simulink model "CompleteModelSimulink"  (R2024a)
settings: Solver=ode45  StartTime=0.0  StopTime=endtime  RelTol=1e-3
values from neighbouring files (symbols this model uses):
  D = 0.069    [CompleteModel.m]
  D_H = 2    [PID_Current.m]    (also in PID_NoCurrent.m = 1)
  D_X = 2    [PID_Current.m]    (also in PID_NoCurrent.m = 1.05)
  D_Y = 2    [PID_Current.m]    (also in PID_NoCurrent.m = 0.8)
  DC =     [DC.mat]
  I_H = 0.1    [PID_Current.m]    (also in PID_NoCurrent.m = 0.01)
  I_X = 0.1    [PID_Current.m]    (also in PID_NoCurrent.m = 0.001)
  I_Y = 0.2    [PID_Current.m]    (also in PID_NoCurrent.m = 0.01)
  InitialPos = [0;0;0]    [CompleteModel.m]
  M_matrix = [2.5 0 0; 0 2.50 0; 0 0 1]    [CompleteModel.m]
  P_H = 2    [PID_Current.m]    (also in PID_NoCurrent.m = 1)
  P_X = 2    [PID_Current.m]    (also in PID_NoCurrent.m = 0.75)
  P_Y = 2    [PID_Current.m]    (also in PID_NoCurrent.m = 1.3)
  Ref = [1;0;0]    [CompleteModel.m]
  SpeedFactor = 0.07    [CompleteModel.m]
  SR =     [SR.mat]
  T_matrix = [0 1 0; 1 0 1; 0.35 -0.065 -0.35]    [CompleteModel.m]
  TauE = [-0.15;0;0]    [CompleteModel.m]
libraries: slpidlib x8
(part 2 of 2)

== system CompleteModelSimulink/Starboard Azimith Thrust generation/Motor+Control SB/Current Controller ==
  Ia : Inport
  Ia ref* : Inport  Port=2
  Constant : Constant  Value=DC.Irated
  Divide : Product  Inputs=*/
  Error : Sum  Inputs=|+-
  PID Controller : slpidlib/PID Controller  Controller=PID  Form=Ideal  TimeDomain=Continuous-time  UseExternalTs=off  SampleTime=-1  IntegratorMethod=Forward Euler  FilterMethod=Forward Euler  ControllerParametersSource=internal  P=7.2353580328522  I=2.78600690342995  UseKiTs=off  D=0.0824758010540437  UseExternalDerivativeSource=off  N=135.726193036092  UseFilter=on  TunerSelectOption=Transfer Function Based (PID Tuner App)  InitialConditionSource=internal  InitialConditionForIntegrator=0  InitialConditionForFilter=0  DifferentiatorICPrevScaledInput=0  ExternalReset=none  TrackingMode=off  Kt=1  LimitOutput=off  SatLimitsSource=internal  UpperSaturationLimit=inf  LowerSaturationLimit=-inf  LinearizeAsGain=on  AntiWindupMode=none  Kb=1  LimitIntegrator=off  UpperIntegratorSaturationLimit=inf  LowerIntegratorSaturationLimit=-inf  POutMin=[]  POutMax=[]  IOutMin=[]  IOutMax=[]  DOutMin=[]  DOutMax=[]  NOutMin=[]  NOutMax=[]  SumOutMin=[]  SumOutMax=[]  SaturationOutMin=[]  SaturationOutMax=[]  PParamMin=[]  PParamMax=[]  IParamMin=[]  IParamMax=[]  DParamMin=[]  DParamMax=[]  NParamMin=[]  NParamMax=[]  KbParamMin=[]  KbParamMax=[]  KtParamMin=[]  KtParamMax=[]  KbOutMin=[]  KbOutMax=[]  KtOutMin=[]  KtOutMax=[]  IntegratorOutMin=[]  IntegratorOutMax=[]  FilterOutMin=[]  FilterOutMax=[]  SumI1OutMin=[]  SumI1OutMax=[]  SumI2OutMin=[]  SumI2OutMax=[]  SumI3OutMin=[]  SumI3OutMax=[]  SumI4OutMin=[]  SumI4OutMax=[]  SumDOutMin=[]  SumDOutMax=[]  DifferentiatorOutMin=[]  DifferentiatorOutMax=[]  FilterDiffOutCoefMin=[]  FilterDiffOutCoefMax=[]  ReciprocalOutMin=[]  ReciprocalOutMax=[]  SumDenOutMin=[]  SumDenOutMax=[]  SumNumOutMin=[]  SumNumOutMax=[]  DivideOutMin=[]  DivideOutMax=[]  UdiffTsProdOutMin=[]  UdiffTsProdOutMax=[]  NTsProdOutMin=[]  NTsProdOutMax=[]  UintegralTsProdOutMin=[]  UintegralTsProdOutMax=[]  UngainTsProdOutMin=[]  UngainTsProdOutMax=[]  ClampingZeroOutDataTypeStr=Inherit: Inherit via back propagation  ClampingZeroOutMin=[]  ClampingZeroOutMax=[]  FilterDenConstantOutDataTypeStr=Inherit: Inherit via back propagation  FilterDenConstantOutMin=[]  FilterDenConstantOutMax=[]  PCopyOutDataTypeStr=Inherit: Inherit via back propagation  PCopyOutMin=[]  PCopyOutMax=[]  NCopyOutDataTypeStr=Inherit: Inherit via back propagation  NCopyOutMin=[]  NCopyOutMax=[]  IntegratorContinuousStateAttributes=''  IntegratorStateMustResolveToSignalObject=off  IntegratorRTWStateStorageClass=Auto  FilterContinuousStateAttributes=''  FilterStateMustResolveToSignalObject=off  FilterRTWStateStorageClass=Auto  ParallelPVariant=Passthrough  IdealPVariant=InternalParameters  IVariant=InternalParameters  DVariant=InternalParameters  IntegratorVariant=Continuous  SatVariant=Disabled  AWVariant=Passthrough  PCopyVariant=Disabled  TRVariant=Disabled  FdbkBlocksVariant=Forward  IdealPFdbkVariant=Disabled  SatFdbkVariant=Disabled  DerivativeFilterVariant=ContFilter  NVariant=InternalParameters  NCopyVariant=Disabled  FilterICVariant=InternalICsFilter  IntegratorICVariant=InternalICs  ExternalResetVariant=Disabled  TRSumVariant=Passthrough  SumFdbkVariant=Disabled  SumVariant=Sum_PID  TsampFilterVariant=InternalTs  TsampNgainVariant=Passthrough  TsampIntegralVariant=Disabled_SignalSpec  ExternalSaturationOutDataTypeStr=Inherit: Same as second input  DerivativeSourceVariant=ErrorSignal
  PID Controller1 : slpidlib/PID Controller  Commented=on  Controller=PID  Form=Ideal  TimeDomain=Continuous-time  UseExternalTs=off  SampleTime=-1  IntegratorMethod=Forward Euler  FilterMethod=Forward Euler  ControllerParametersSource=internal  P=7.2353580328522  I=2.78600690342995  UseKiTs=off  D=0.0824758010540437  UseExternalDerivativeSource=off  N=135.726193036092  UseFilter=on  TunerSelectOption=Transfer Function Based (PID Tuner App)  InitialConditionSource=internal  InitialConditionForIntegrator=0  InitialConditionForFilter=0  DifferentiatorICPrevScaledInput=0  ExternalReset=none  TrackingMode=off  Kt=1  LimitOutput=off  SatLimitsSource=internal  UpperSaturationLimit=inf  LowerSaturationLimit=-inf  LinearizeAsGain=on  AntiWindupMode=none  Kb=1  LimitIntegrator=off  UpperIntegratorSaturationLimit=inf  LowerIntegratorSaturationLimit=-inf  POutMin=[]  POutMax=[]  IOutMin=[]  IOutMax=[]  DOutMin=[]  DOutMax=[]  NOutMin=[]  NOutMax=[]  SumOutMin=[]  SumOutMax=[]  SaturationOutMin=[]  SaturationOutMax=[]  PParamMin=[]  PParamMax=[]  IParamMin=[]  IParamMax=[]  DParamMin=[]  DParamMax=[]  NParamMin=[]  NParamMax=[]  KbParamMin=[]  KbParamMax=[]  KtParamMin=[]  KtParamMax=[]  KbOutMin=[]  KbOutMax=[]  KtOutMin=[]  KtOutMax=[]  IntegratorOutMin=[]  IntegratorOutMax=[]  FilterOutMin=[]  FilterOutMax=[]  SumI1OutMin=[]  SumI1OutMax=[]  SumI2OutMin=[]  SumI2OutMax=[]  SumI3OutMin=[]  SumI3OutMax=[]  SumI4OutMin=[]  SumI4OutMax=[]  SumDOutMin=[]  SumDOutMax=[]  DifferentiatorOutMin=[]  DifferentiatorOutMax=[]  FilterDiffOutCoefMin=[]  FilterDiffOutCoefMax=[]  ReciprocalOutMin=[]  ReciprocalOutMax=[]  SumDenOutMin=[]  SumDenOutMax=[]  SumNumOutMin=[]  SumNumOutMax=[]  DivideOutMin=[]  DivideOutMax=[]  UdiffTsProdOutMin=[]  UdiffTsProdOutMax=[]  NTsProdOutMin=[]  NTsProdOutMax=[]  UintegralTsProdOutMin=[]  UintegralTsProdOutMax=[]  UngainTsProdOutMin=[]  UngainTsProdOutMax=[]  ClampingZeroOutDataTypeStr=Inherit: Inherit via back propagation  ClampingZeroOutMin=[]  ClampingZeroOutMax=[]  FilterDenConstantOutDataTypeStr=Inherit: Inherit via back propagation  FilterDenConstantOutMin=[]  FilterDenConstantOutMax=[]  PCopyOutDataTypeStr=Inherit: Inherit via back propagation  PCopyOutMin=[]  PCopyOutMax=[]  NCopyOutDataTypeStr=Inherit: Inherit via back propagation  NCopyOutMin=[]  NCopyOutMax=[]  IntegratorContinuousStateAttributes=''  IntegratorStateMustResolveToSignalObject=off  IntegratorRTWStateStorageClass=Auto  FilterContinuousStateAttributes=''  FilterStateMustResolveToSignalObject=off  FilterRTWStateStorageClass=Auto  ParallelPVariant=Passthrough  IdealPVariant=InternalParameters  IVariant=InternalParameters  DVariant=InternalParameters  IntegratorVariant=Continuous  SatVariant=Disabled  AWVariant=Passthrough  PCopyVariant=Disabled  TRVariant=Disabled  FdbkBlocksVariant=Forward  IdealPFdbkVariant=Disabled  SatFdbkVariant=Disabled  DerivativeFilterVariant=ContFilter  NVariant=InternalParameters  NCopyVariant=Disabled  FilterICVariant=InternalICsFilter  IntegratorICVariant=InternalICs  ExternalResetVariant=Disabled  TRSumVariant=Passthrough  SumFdbkVariant=Disabled  SumVariant=Sum_PID  TsampFilterVariant=InternalTs  TsampNgainVariant=Passthrough  TsampIntegralVariant=Disabled_SignalSpec  ExternalSaturationOutDataTypeStr=Inherit: Same as second input  DerivativeSourceVariant=ErrorSignal
  Saturation : Saturate  UpperLimit=1.2*DC.Irated  LowerLimit=-0.5*DC.Irated
  Ia ref : Outport
  wires:
  Error/1 -> Divide/1
  Divide/1 -> PID Controller/1
  PID Controller/1 -> Saturation/1
  Ia/1 -> Error/2
  Saturation/1 -> Ia ref/1
  Ia ref*/1 -> Error/1
  Constant/1 -> Divide/2

== system CompleteModelSimulink/Starboard Azimith Thrust generation/Motor+Control SB/Motor system ==
  Terminal Voltage : Inport
  Mechnical Torque : Inport  Port=2
  Electrical Equation : Subsystem
  Mechnical Equation : Subsystem
  Ia : Outport
  Wm1 : Outport  Port=2
  wires:
  Electrical Equation/1(Ia) -> Ia/1, Mechnical Equation/1(Ia)
  Mechnical Torque/1 -> Mechnical Equation/2(Mechnical Torque)
  Terminal Voltage/1 -> Electrical Equation/1(Terminal Voltage)
  Mechnical Equation/1(Wm) -> Wm1/1, Electrical Equation/2(Wm)

== system CompleteModelSimulink/Starboard Azimith Thrust generation/Motor+Control SB/Speed control ==
  Ref speed : Inport
  Act speed : Inport  Port=2
  Constant : Constant  Value=DC.Omegarated
  Divide : Product  Inputs=/*
  PID Controller2 : slpidlib/PID Controller  Controller=PID  Form=Ideal  TimeDomain=Continuous-time  UseExternalTs=off  SampleTime=-1  IntegratorMethod=Forward Euler  FilterMethod=Forward Euler  ControllerParametersSource=internal  P=301.958567368747  I=2.49617195964231  UseKiTs=off  D=0.0354093832005891  UseExternalDerivativeSource=off  N=1725.20945072566  UseFilter=on  TunerSelectOption=Transfer Function Based (PID Tuner App)  InitialConditionSource=internal  InitialConditionForIntegrator=0  InitialConditionForFilter=0  DifferentiatorICPrevScaledInput=0  ExternalReset=none  TrackingMode=off  Kt=1  LimitOutput=off  SatLimitsSource=internal  UpperSaturationLimit=inf  LowerSaturationLimit=-inf  LinearizeAsGain=on  AntiWindupMode=none  Kb=1  LimitIntegrator=off  UpperIntegratorSaturationLimit=inf  LowerIntegratorSaturationLimit=-inf  POutMin=[]  POutMax=[]  IOutMin=[]  IOutMax=[]  DOutMin=[]  DOutMax=[]  NOutMin=[]  NOutMax=[]  SumOutMin=[]  SumOutMax=[]  SaturationOutMin=[]  SaturationOutMax=[]  PParamMin=[]  PParamMax=[]  IParamMin=[]  IParamMax=[]  DParamMin=[]  DParamMax=[]  NParamMin=[]  NParamMax=[]  KbParamMin=[]  KbParamMax=[]  KtParamMin=[]  KtParamMax=[]  KbOutMin=[]  KbOutMax=[]  KtOutMin=[]  KtOutMax=[]  IntegratorOutMin=[]  IntegratorOutMax=[]  FilterOutMin=[]  FilterOutMax=[]  SumI1OutMin=[]  SumI1OutMax=[]  SumI2OutMin=[]  SumI2OutMax=[]  SumI3OutMin=[]  SumI3OutMax=[]  SumI4OutMin=[]  SumI4OutMax=[]  SumDOutMin=[]  SumDOutMax=[]  DifferentiatorOutMin=[]  DifferentiatorOutMax=[]  FilterDiffOutCoefMin=[]  FilterDiffOutCoefMax=[]  ReciprocalOutMin=[]  ReciprocalOutMax=[]  SumDenOutMin=[]  SumDenOutMax=[]  SumNumOutMin=[]  SumNumOutMax=[]  DivideOutMin=[]  DivideOutMax=[]  UdiffTsProdOutMin=[]  UdiffTsProdOutMax=[]  NTsProdOutMin=[]  NTsProdOutMax=[]  UintegralTsProdOutMin=[]  UintegralTsProdOutMax=[]  UngainTsProdOutMin=[]  UngainTsProdOutMax=[]  ClampingZeroOutDataTypeStr=Inherit: Inherit via back propagation  ClampingZeroOutMin=[]  ClampingZeroOutMax=[]  FilterDenConstantOutDataTypeStr=Inherit: Inherit via back propagation  FilterDenConstantOutMin=[]  FilterDenConstantOutMax=[]  PCopyOutDataTypeStr=Inherit: Inherit via back propagation  PCopyOutMin=[]  PCopyOutMax=[]  NCopyOutDataTypeStr=Inherit: Inherit via back propagation  NCopyOutMin=[]  NCopyOutMax=[]  IntegratorContinuousStateAttributes=''  IntegratorStateMustResolveToSignalObject=off  IntegratorRTWStateStorageClass=Auto  FilterContinuousStateAttributes=''  FilterStateMustResolveToSignalObject=off  FilterRTWStateStorageClass=Auto  ParallelPVariant=Passthrough  IdealPVariant=InternalParameters  IVariant=InternalParameters  DVariant=InternalParameters  IntegratorVariant=Continuous  SatVariant=Disabled  AWVariant=Passthrough  PCopyVariant=Disabled  TRVariant=Disabled  FdbkBlocksVariant=Forward  IdealPFdbkVariant=Disabled  SatFdbkVariant=Disabled  DerivativeFilterVariant=ContFilter  NVariant=InternalParameters  NCopyVariant=Disabled  FilterICVariant=InternalICsFilter  IntegratorICVariant=InternalICs  ExternalResetVariant=Disabled  TRSumVariant=Passthrough  SumFdbkVariant=Disabled  SumVariant=Sum_PID  TsampFilterVariant=InternalTs  TsampNgainVariant=Passthrough  TsampIntegralVariant=Disabled_SignalSpec  ExternalSaturationOutDataTypeStr=Inherit: Same as second input  DerivativeSourceVariant=ErrorSignal
  Saturation : Saturate  UpperLimit=1.2*DC.Irated  LowerLimit=-0.5*DC.Irated
  Sum : Sum  Inputs=|+-
  Ia ref* : Outport
  wires:
  Saturation/1 -> Ia ref*/1
  PID Controller2/1 -> Saturation/1
  Divide/1 -> PID Controller2/1
  Ref speed/1 -> Sum/1
  Act speed/1 -> Sum/2
  Sum/1 -> Divide/2  "Error"
  Constant/1 -> Divide/1

== system CompleteModelSimulink/Vessel reaction to forces/Rotate local to global /Local to global x  ==
  X : Inport
  Y : Inport  Port=2
  theta : Inport  Port=3
  Add : Sum
  Product : Product
  Product1 : Product
  Trigonometric Function : Trigonometry  Operator=cos
  Trigonometric Function1 : Trigonometry
  x : Outport  VectorParamsAs1DForOutWhenUnconnected=off
  wires:
  Add/1 -> x/1
  Product1/1 -> Add/2
  Product/1 -> Add/1
  Y/1 -> Product1/1
  X/1 -> Product/1
  theta/1 -> Trigonometric Function1/1, Trigonometric Function/1
  Trigonometric Function1/1 -> Product1/2
  Trigonometric Function/1 -> Product/2

== system CompleteModelSimulink/Vessel reaction to forces/Rotate local to global /Local to global y ==
  X : Inport
  Y : Inport  Port=2
  theta : Inport  Port=3
  Product : Product
  Product1 : Product
  Sum : Sum  Inputs=-+
  Trigonometric Function : Trigonometry
  Trigonometric Function1 : Trigonometry  Operator=cos
  y : Outport  VectorParamsAs1DForOutWhenUnconnected=off
  wires:
  Sum/1 -> y/1
  Product1/1 -> Sum/2
  Y/1 -> Product1/1
  X/1 -> Product/1
  theta/1 -> Trigonometric Function1/1, Trigonometric Function/1
  Trigonometric Function1/1 -> Product1/2
  Trigonometric Function/1 -> Product/2
  Product/1 -> Sum/1

== system CompleteModelSimulink/Portside Azimuth Thrust generation/Motor+Control PS/Motor system/Electrical Equation ==
  Terminal Voltage : Inport
  Wm : Inport  Port=2
  I : Integrator
  Kt*wm : Gain  Gain=DC.Kb
  La*didt : Sum  Inputs=+--
  Ra*Ia : Gain  Gain=DC.Ra
  didt : Gain  Gain=1/DC.La
  Ia : Outport
  wires:
  Wm/1 -> Kt*wm/1
  Kt*wm/1 -> La*didt/2
  didt/1 -> I/1
  Terminal Voltage/1 -> La*didt/1
  La*didt/1 -> didt/1
  Ra*Ia/1 -> La*didt/3
  I/1 -> Ra*Ia/1, Ia/1

== system CompleteModelSimulink/Portside Azimuth Thrust generation/Motor+Control PS/Motor system/Mechnical Equation ==
  Ia : Inport
  Mechnical Torque : Inport  Port=2
  Cm*wm : Gain  Gain=DC.Cm
  Jm* dwdt : Sum  Inputs=-+-
  Kt*Ia : Gain  Gain=DC.Kt
  dwdt : Gain  Gain=1/DC.Jm
  wm : Integrator
  Wm : Outport
  wires:
  wm/1 -> Cm*wm/1, Wm/1
  dwdt/1 -> wm/1
  Mechnical Torque/1 -> Jm* dwdt/3
  Cm*wm/1 -> Jm* dwdt/1
  Jm* dwdt/1 -> dwdt/1
  Ia/1 -> Kt*Ia/1
  Kt*Ia/1 -> Jm* dwdt/2

== system CompleteModelSimulink/Starboard Azimith Thrust generation/Motor+Control SB/Motor system/Electrical Equation ==
  Terminal Voltage : Inport
  Wm : Inport  Port=2
  I : Integrator
  Kt*wm : Gain  Gain=DC.Kb
  La*didt : Sum  Inputs=+--
  Ra*Ia : Gain  Gain=DC.Ra
  didt : Gain  Gain=1/DC.La
  Ia : Outport
  wires:
  Wm/1 -> Kt*wm/1
  Kt*wm/1 -> La*didt/2
  didt/1 -> I/1
  Terminal Voltage/1 -> La*didt/1
  La*didt/1 -> didt/1
  Ra*Ia/1 -> La*didt/3
  I/1 -> Ra*Ia/1, Ia/1

== system CompleteModelSimulink/Starboard Azimith Thrust generation/Motor+Control SB/Motor system/Mechnical Equation ==
  Ia : Inport
  Mechnical Torque : Inport  Port=2
  Cm*wm : Gain  Gain=DC.Cm
  Jm* dwdt : Sum  Inputs=-+-
  Kt*Ia : Gain  Gain=DC.Kt
  dwdt : Gain  Gain=1/DC.Jm
  wm : Integrator
  Wm : Outport
  wires:
  wm/1 -> Cm*wm/1, Wm/1
  dwdt/1 -> wm/1
  Mechnical Torque/1 -> Jm* dwdt/3
  Cm*wm/1 -> Jm* dwdt/1
  Jm* dwdt/1 -> dwdt/1
  Ia/1 -> Kt*Ia/1
  Kt*Ia/1 -> Jm* dwdt/2

== matlab function CompleteModelSimulink/Vessel reaction to forces/Corriolis Matrix/MATLAB Function1 ==
  data: uv input; C output; Xudot input; Yvdot input; m input
function C = fcn(uv, Xudot, Yvdot, m)
a1 = Xudot*uv(1);
a2 = Yvdot*uv(2);

Ca = [0 0 a2; 0 0 -a1; -a2 a1 0];

Crb = [0 0 -m*uv(2); 0 0 m*uv(1); m*uv(2) -m*uv(1) 0];

C = Ca+Crb;

== matlab function CompleteModelSimulink/Vessel reaction to forces/Damping Vector/Damping ==
  data: uvr input; D output; X input; Y input; Yaw input; L input
function D = fcn(uvr, X, Y, Yaw, L)
    D11 = X(1)*uvr(1)^3+X(2)*uvr(1)^2+X(3)*uvr(1)+X(4);
    D22 = Y(1)*uvr(2)^3+Y(2)*uvr(2)^2+Y(3)*uvr(2)+Y(4);
    D33 = 1/80*Yaw(1)*uvr(3)^3*L^4+1/12*Yaw(2)*L^2*uvr(3);
D = [D11;D22;D33];

== matlab function CompleteModelSimulink/Portside Azimuth Thrust generation/Thrust to Torque/Matching PS ==
  data: Kt input; Kq output
function Kq = fcn(Kt)
coef = [-14.707 5.8681 -4.0985 1.5002];
J = coef(1)*Kt^3+coef(2)*Kt^2+coef(3)*Kt+coef(4);
coef2 = [0.038 -0.0158 -0.0178 0.0513];
Kq = coef2(1)*J^3+coef2(2)*J^2+coef2(3)*J+coef2(4);

== matlab function CompleteModelSimulink/Starboard Azimith Thrust generation/Trust to Torque1/Matching PS ==
  data: Kt input; Kq output
function Kq = fcn(Kt)
coef = [-14.707 5.8681 -4.0985 1.5002];
J = coef(1)*Kt^3+coef(2)*Kt^2+coef(3)*Kt+coef(4);
coef2 = [0.038 -0.0158 -0.0178 0.0513];
Kq = coef2(1)*J^3+coef2(2)*J^2+coef2(3)*J+coef2(4);

== matlab function CompleteModelSimulink/Current force handler/Current Forces/Damping ==
  data: uvr input; D output; X input; Y input; Yaw input; L input
function D = fcn(uvr, X, Y, Yaw, L)
    D11 = X(1)*uvr(1)^3+X(2)*uvr(1)^2+X(3)*uvr(1)+X(4);
    D22 = Y(1)*uvr(2)^3+Y(2)*uvr(2)^2+Y(3)*uvr(2)+Y(4);
    D33 = 1/80*Yaw(1)*uvr(3)^3*L^4+1/12*Yaw(2)*L^2*uvr(3);
D = [D11;D22;D33];
